simulink model "quad_control_elev8_attit_training"  (Simulink 8.7)
settings: Solver=FixedStepAuto  StartTime=0.0  StopTime=10  FixedStep=0.01  RelTol=1e-3
InitFcn:
  | % --- Inner loop gains --------
  | %Kp_pitch= 2.5; I_pitch =0.005; D_pitch = 0.5;
  | %Kp_roll = 2.5; I_roll =0.005; D_roll = 0.5;
  | %Kp_yaw = 10; I_yaw = 0.003; D_yaw = 2;
  | % --------------------------
  | 
  | % --- Outer loop gains --------
  | P_Z = 26.3889;
  | I_Z = 22.8237;
  | D_Z = 20.4994;
  | % --------------------------
  | 
  | % --- Saturation limits --------
  | mvel_upper_limit = 50;
  | mvel_lower_limit = 0;
  | % --------------------------
  | 
  | global clientID;
  | clientID=-1;
values from neighbouring files (symbols this model uses):
  D_pitch = 0.883609617998    [workspace_inner.mat]
  D_roll = 0.689579833659    [workspace_inner.mat]
  D_yaw = 2.7680176295    [workspace_inner.mat]
  I_pitch = 0.0103644908387    [workspace_inner.mat]
  I_roll = 0.00715888678063    [workspace_inner.mat]
  I_yaw = 0.00215447703315    [workspace_inner.mat]
  Kp_pitch = 3.99957984924    [workspace_inner.mat]
  Kp_roll = 4.19505963961    [workspace_inner.mat]
  Kp_yaw = 8.12783574482    [workspace_inner.mat]
undefined symbols (not defined in the file or in its folder): Angular, Linear
libraries: robotlib x7, simulink_extras x6, aerolibtransform2 x2
settings Model: Creator=kleber  LastModifiedBy=kleber
settings DebuggingCC: UnderspecifiedInitializationDetection=Simplified  MergeDetectMultiDrivingBlocksExec=error  SolverPrmCheckMsg=warning
settings ConfigComp: CovSFcnEnable=off

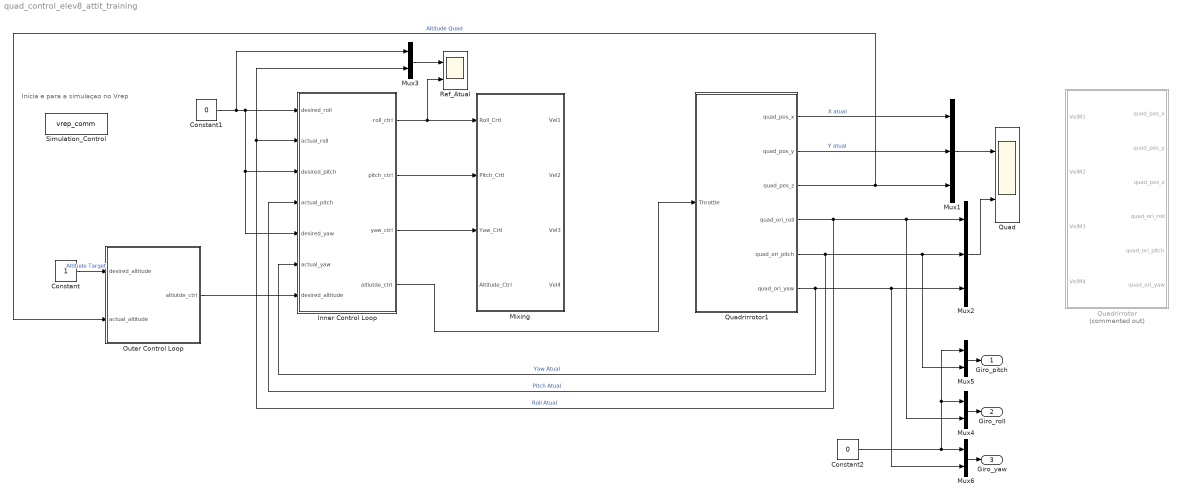
== system quad_control_elev8_attit_training ==
  note: Inicia e para a simulaçao no Vrep
  Constant : Constant
  Constant1 : Constant  Value=0
  Constant2 : Constant  Value=0
  Inner Control Loop : Subsystem
  Mixing : Subsystem
  Mux1 : Mux  Inputs=3
  Mux2 : Mux  Inputs=3
  Mux{3..6} (4 alike) : Mux  Inputs=2
  Outer Control Loop : Subsystem
  Quad : Scope  NumInputPorts=2
  Quadrirrotor : Subsystem  Commented=on
  Quadrirrotor1 : Subsystem
  Ref_Atual : Scope  NumInputPorts=2
  Simulation_Control : S-Function  FunctionName=vrep_comm  SFunctionDeploymentMode=off  EnableBusSupport=off
  Giro_pitch : Outport
  Giro_roll : Outport  Port=2
  Giro_yaw : Outport  Port=3
  wires:
  Mux1/1 -> Quad/1
  Mux2/1 -> Quad/2
  Quadrirrotor1/5(quad_ori_pitch) -> Mux2/2, Mux5/2, Inner Control Loop/4(actual_pitch)  "Pitch Atual"
  Quadrirrotor1/4(quad_ori_roll) -> Mux2/1, Mux4/2, Inner Control Loop/2(actual_roll), Mux3/2  "Roll Atual"
  Quadrirrotor1/1(quad_pos_x) -> Mux1/1  "X atual"
  Quadrirrotor1/3(quad_pos_z) -> Mux1/3, Outer Control Loop/2(actual_altitude)  "Altitude Quad"
  Quadrirrotor1/6(quad_ori_yaw) -> Mux6/2, Mux2/3, Inner Control Loop/6(actual_yaw)  "Yaw Atual"
  Inner Control Loop/4(altiutde_ctrl) -> Quadrirrotor1/1(Throttle)
  Constant1/1 -> Inner Control Loop/1(desired_roll), Inner Control Loop/5(desired_yaw), Inner Control Loop/3(desired_pitch), Mux3/1
  Outer Control Loop/1(altiutde_ctrl) -> Inner Control Loop/7(desired_altitude)
  Quadrirrotor1/2(quad_pos_y) -> Mux1/2  "Y atual"
  Constant/1 -> Outer Control Loop/1(desired_altitude)  "Altitude Target"
  Mux3/1 -> Ref_Atual/1
  Mux4/1 -> Giro_roll/1
  Mux5/1 -> Giro_pitch/1
  Mux6/1 -> Giro_yaw/1
  Constant2/1 -> Mux6/1, Mux4/1, Mux5/1
  Inner Control Loop/1(roll_ctrl) -> Ref_Atual/2, Mixing/1(Roll_Crtl)
  Inner Control Loop/2(pitch_ctrl) -> Mixing/2(Pitch_Crtl)
  Inner Control Loop/3(yaw_ctrl) -> Mixing/3(Yaw_Crtl)

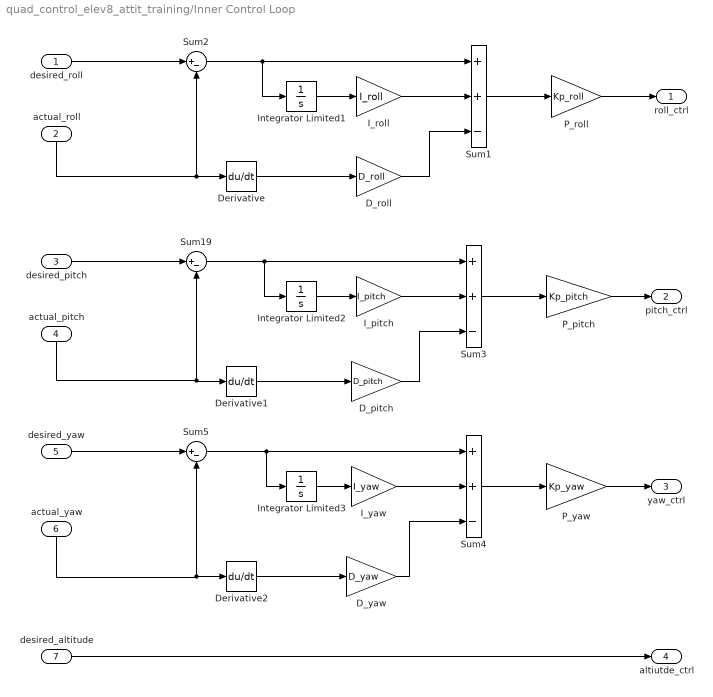
== system quad_control_elev8_attit_training/Inner Control Loop ==
  desired_roll : Inport
  actual_roll : Inport  Port=2
  desired_pitch : Inport  Port=3
  actual_pitch : Inport  Port=4
  desired_yaw : Inport  Port=5
  actual_yaw : Inport  Port=6
  desired_altitude : Inport  Port=7
  D_pitch : Gain  Gain=D_pitch
  D_roll : Gain  Gain=D_roll
  D_yaw : Gain  Gain=D_yaw
  Derivative : Derivative
  Derivative1 : Derivative
  Derivative2 : Derivative
  I_pitch : Gain  Gain=I_pitch
  I_roll : Gain  Gain=I_roll
  I_yaw : Gain  Gain=I_yaw
  Integrator Limited1 : Integrator  LimitOutput=on  UpperSaturationLimit=100  LowerSaturationLimit=-100
  Integrator Limited2 : Integrator  LimitOutput=on  UpperSaturationLimit=100  LowerSaturationLimit=-100
  Integrator Limited3 : Integrator  LimitOutput=on  UpperSaturationLimit=100  LowerSaturationLimit=-100
  P_pitch : Gain  Gain=Kp_pitch
  P_roll : Gain  Gain=Kp_roll
  P_yaw : Gain  Gain=Kp_yaw
  Sum1 : Sum  Inputs=++-
  Sum19 : Sum  Inputs=|+-
  Sum2 : Sum  Inputs=|+-
  Sum3 : Sum  Inputs=++-
  Sum4 : Sum  Inputs=++-
  Sum5 : Sum  Inputs=|+-
  roll_ctrl : Outport
  pitch_ctrl : Outport  Port=2
  yaw_ctrl : Outport  Port=3
  altiutde_ctrl : Outport  Port=4
  wires:
  desired_altitude/1 -> altiutde_ctrl/1
  Sum3/1 -> P_pitch/1
  P_pitch/1 -> pitch_ctrl/1
  D_pitch/1 -> Sum3/3
  Derivative1/1 -> D_pitch/1
  actual_pitch/1 -> Sum19/2, Derivative1/1
  Sum2/1 -> Integrator Limited1/1, Sum1/1
  Sum1/1 -> P_roll/1
  D_roll/1 -> Sum1/3
  Derivative/1 -> D_roll/1
  desired_pitch/1 -> Sum19/1
  actual_roll/1 -> Sum2/2, Derivative/1
  desired_roll/1 -> Sum2/1
  actual_yaw/1 -> Sum5/2, Derivative2/1
  Derivative2/1 -> D_yaw/1
  D_yaw/1 -> Sum4/3
  desired_yaw/1 -> Sum5/1
  P_roll/1 -> roll_ctrl/1
  P_yaw/1 -> yaw_ctrl/1
  I_roll/1 -> Sum1/2
  Sum19/1 -> Integrator Limited2/1, Sum3/1
  I_pitch/1 -> Sum3/2
  Sum4/1 -> P_yaw/1
  I_yaw/1 -> Sum4/2
  Integrator Limited2/1 -> I_pitch/1
  Integrator Limited1/1 -> I_roll/1
  Integrator Limited3/1 -> I_yaw/1
  Sum5/1 -> Integrator Limited3/1, Sum4/1

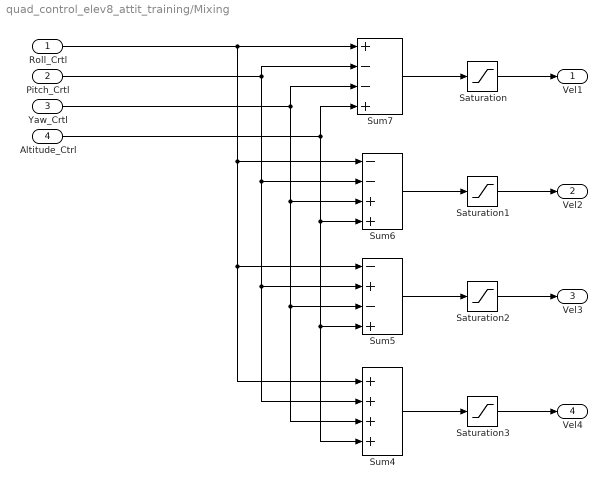
== system quad_control_elev8_attit_training/Mixing ==
  Roll_Crtl : Inport
  Pitch_Crtl : Inport  Port=2
  Yaw_Crtl : Inport  Port=3
  Altitude_Ctrl : Inport  Port=4
  Saturation{,1..3} (4 alike) : Saturate  UpperLimit=mvel_upper_limit  LowerLimit=mvel_lower_limit
  Sum4 : Sum  Inputs=++++
  Sum5 : Sum  Inputs=-+-+
  Sum6 : Sum  Inputs=--++
  Sum7 : Sum  Inputs=+--+
  Vel1 : Outport
  Vel2 : Outport  Port=2
  Vel3 : Outport  Port=3
  Vel4 : Outport  Port=4
  wires:
  Yaw_Crtl/1 -> Sum4/3, Sum5/3, Sum6/3, Sum7/3
  Roll_Crtl/1 -> Sum4/1, Sum5/1, Sum6/1, Sum7/1
  Pitch_Crtl/1 -> Sum4/2, Sum5/2, Sum6/2, Sum7/2
  Altitude_Ctrl/1 -> Sum4/4, Sum5/4, Sum6/4, Sum7/4
  Sum7/1 -> Saturation/1
  Saturation/1 -> Vel1/1
  Sum6/1 -> Saturation1/1
  Saturation1/1 -> Vel2/1
  Sum5/1 -> Saturation2/1
  Saturation2/1 -> Vel3/1
  Sum4/1 -> Saturation3/1
  Saturation3/1 -> Vel4/1

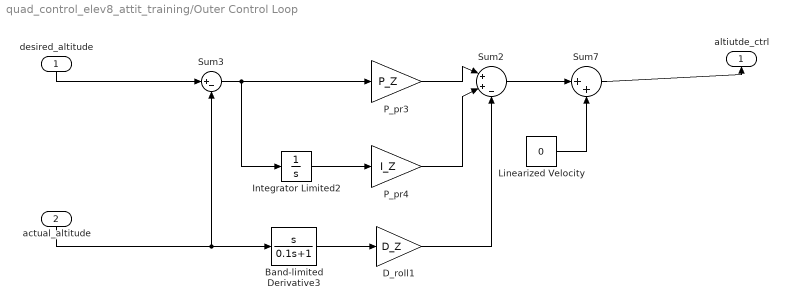
== system quad_control_elev8_attit_training/Outer Control Loop ==
  desired_altitude : Inport
  actual_altitude : Inport  Port=2
  Band-limited Derivative3 : TransferFcn  Numerator=[1 0]  Denominator=[0.1 1]
  D_roll1 : Gain  Gain=D_Z
  Integrator Limited2 : Integrator  LimitOutput=on  UpperSaturationLimit=5  LowerSaturationLimit=0
  Linearized Velocity : Constant  Value=0
  P_pr3 : Gain  Gain=P_Z
  P_pr4 : Gain  Gain=I_Z
  Sum2 : Sum  Inputs=|++-
  Sum3 : Sum  Inputs=|+-
  Sum7 : Sum  Inputs=|++
  altiutde_ctrl : Outport
  wires:
  Sum3/1 -> Integrator Limited2/1, P_pr3/1
  Integrator Limited2/1 -> P_pr4/1
  P_pr3/1 -> Sum2/1
  P_pr4/1 -> Sum2/2
  D_roll1/1 -> Sum2/3
  actual_altitude/1 -> Sum3/2, Band-limited Derivative3/1
  Band-limited Derivative3/1 -> D_roll1/1
  Sum2/1 -> Sum7/1
  Linearized Velocity/1 -> Sum7/2
  desired_altitude/1 -> Sum3/1
  Sum7/1 -> altiutde_ctrl/1

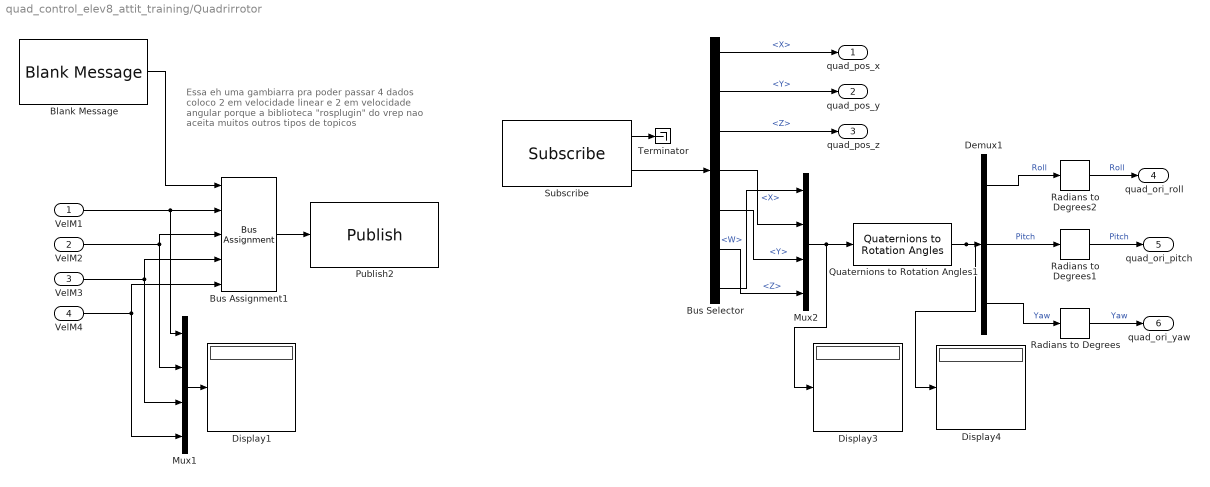
== system quad_control_elev8_attit_training/Quadrirrotor ==
  note: Essa eh uma gambiarra pra poder passar 4 dados coloco 2 em velocidade linear e 2 em velocidade angular porque a biblioteca "rosplugin" do vrep nao aceita muitos outros tipos de topicos
  VelM1 : Inport
  VelM2 : Inport  Port=2
  VelM3 : Inport  Port=3
  VelM4 : Inport  Port=4
  Blank Message : robotlib/Blank Message  SourceLibraryInfo=This block requires Robotics System Toolbox  messageType=geometry_msgs/Twist  SampleTime=inf
  Bus Assignment1 : BusAssignment  DialogController=Simulink.DDGSource_BusAssignment  AssignedSignals=Linear.X,Linear.Y,Angular.X,Angular.Y
  Bus Selector : BusSelector  OutputSignals=Pose.Position.X,Pose.Position.Y,Pose.Position.Z,Pose.Orientation.X,Pose.Orientation.Y,Pose.Orientation.Z,Pose.Orientation.W
  Demux1 : Demux  Outputs=3
  Display1 : Display
  Display3 : Display
  Display4 : Display
  Mux1 : Mux
  Mux2 : Mux
  Publish2 : robotlib/Publish  SourceLibraryInfo=This block requires Robotics System Toolbox  topicSource=Select from ROS network  topic=/motor_velocities  messageType=geometry_msgs/Twist  messageQueueLength=105
  Quaternions to Rotation Angles1 : aerolibtransform2/Quaternions to Rotation Angles  rotationOrder=XYZ
  Radians to Degrees : simulink_extras/Transformations/Radians to Degrees
  Radians to Degrees1 : simulink_extras/Transformations/Radians to Degrees
  Radians to Degrees2 : simulink_extras/Transformations/Radians to Degrees
  Subscribe : robotlib/Subscribe  SourceLibraryInfo=This block requires Robotics System Toolbox  topicSource=Select from ROS network  topic=/quad_pos_ang  messageType=geometry_msgs/PoseStamped  sampleTime=-1  messageQueueLength=51
  Terminator : Terminator
  quad_pos_x : Outport
  quad_pos_y : Outport  Port=2
  quad_pos_z : Outport  Port=3
  quad_ori_roll : Outport  Port=4
  quad_ori_pitch : Outport  Port=5
  quad_ori_yaw : Outport  Port=6
  wires:
  VelM1/1 -> Mux1/1, Bus Assignment1/2
  Bus Selector/1 -> quad_pos_x/1  "<X>"
  Bus Selector/2 -> quad_pos_y/1  "<Y>"
  Bus Selector/3 -> quad_pos_z/1  "<Z>"
  Radians to Degrees2/1 -> quad_ori_roll/1  "Roll"
  Radians to Degrees1/1 -> quad_ori_pitch/1  "Pitch"
  Radians to Degrees/1 -> quad_ori_yaw/1  "Yaw"
  Demux1/3 -> Radians to Degrees/1  "Yaw"
  Demux1/2 -> Radians to Degrees1/1  "Pitch"
  Demux1/1 -> Radians to Degrees2/1  "Roll"
  Bus Assignment1/1 -> Publish2/1
  Blank Message/1 -> Bus Assignment1/1
  Subscribe/2 -> Bus Selector/1
  Subscribe/1 -> Terminator/1
  Mux2/1 -> Quaternions to Rotation Angles1/1, Display3/1
  Bus Selector/5 -> Mux2/3  "<Y>"
  Bus Selector/6 -> Mux2/4  "<Z>"
  Bus Selector/7 -> Mux2/1  "<W>"
  Quaternions to Rotation Angles1/1 -> Demux1/1, Display4/1
  Bus Selector/4 -> Mux2/2  "<X>"
  VelM2/1 -> Bus Assignment1/3, Mux1/2
  VelM3/1 -> Bus Assignment1/4, Mux1/3
  VelM4/1 -> Bus Assignment1/5, Mux1/4
  Mux1/1 -> Display1/1

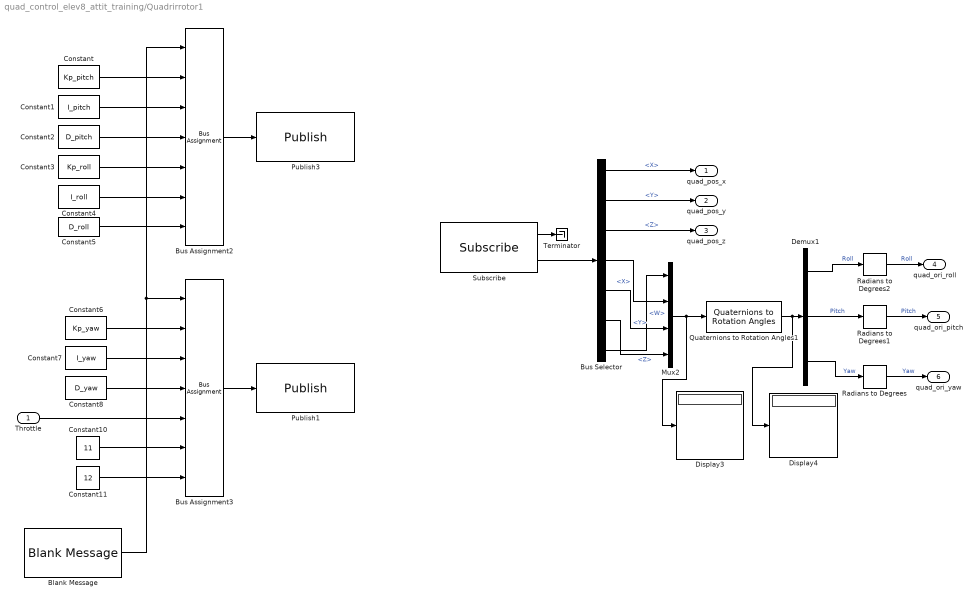
== system quad_control_elev8_attit_training/Quadrirrotor1 ==
  Throttle : Inport
  Blank Message : robotlib/Blank Message  SourceLibraryInfo=This block requires Robotics System Toolbox  messageType=geometry_msgs/Twist  SampleTime=inf
  Bus Assignment2 : BusAssignment  DialogController=Simulink.DDGSource_BusAssignment  AssignedSignals=Linear.X,Linear.Y,Linear.Z,Angular.X,Angular.Y,Angular.Z
  Bus Assignment3 : BusAssignment  DialogController=Simulink.DDGSource_BusAssignment  AssignedSignals=Linear.X,Linear.Y,Linear.Z,Angular.X,Angular.Y,Angular.Z
  Bus Selector : BusSelector  OutputSignals=Pose.Position.X,Pose.Position.Y,Pose.Position.Z,Pose.Orientation.X,Pose.Orientation.Y,Pose.Orientation.Z,Pose.Orientation.W
  Constant : Constant  Value=Kp_pitch
  Constant1 : Constant  Value=I_pitch
  Constant10 : Constant  Value=11
  Constant11 : Constant  Value=12
  Constant2 : Constant  Value=D_pitch
  Constant3 : Constant  Value=Kp_roll
  Constant4 : Constant  Value=I_roll
  Constant5 : Constant  Value=D_roll
  Constant6 : Constant  Value=Kp_yaw
  Constant7 : Constant  Value=I_yaw
  Constant8 : Constant  Value=D_yaw
  Demux1 : Demux  Outputs=3
  Display3 : Display
  Display4 : Display
  Mux2 : Mux
  Publish1 : robotlib/Publish  SourceLibraryInfo=This block requires Robotics System Toolbox  topicSource=Select from ROS network  topic=/gains2  messageType=geometry_msgs/Twist  messageQueueLength=105
  Publish3 : robotlib/Publish  SourceLibraryInfo=This block requires Robotics System Toolbox  topicSource=Select from ROS network  topic=/gains1  messageType=geometry_msgs/Twist  messageQueueLength=105
  Quaternions to Rotation Angles1 : aerolibtransform2/Quaternions to Rotation Angles  rotationOrder=XYZ
  Radians to Degrees : simulink_extras/Transformations/Radians to Degrees
  Radians to Degrees1 : simulink_extras/Transformations/Radians to Degrees
  Radians to Degrees2 : simulink_extras/Transformations/Radians to Degrees
  Subscribe : robotlib/Subscribe  SourceLibraryInfo=This block requires Robotics System Toolbox  topicSource=Select from ROS network  topic=/quad_pos_ang  messageType=geometry_msgs/PoseStamped  sampleTime=-1  messageQueueLength=51
  Terminator : Terminator
  quad_pos_x : Outport
  quad_pos_y : Outport  Port=2
  quad_pos_z : Outport  Port=3
  quad_ori_roll : Outport  Port=4
  quad_ori_pitch : Outport  Port=5
  quad_ori_yaw : Outport  Port=6
  wires:
  Bus Selector/1 -> quad_pos_x/1  "<X>"
  Bus Selector/2 -> quad_pos_y/1  "<Y>"
  Bus Selector/3 -> quad_pos_z/1  "<Z>"
  Radians to Degrees2/1 -> quad_ori_roll/1  "Roll"
  Radians to Degrees1/1 -> quad_ori_pitch/1  "Pitch"
  Radians to Degrees/1 -> quad_ori_yaw/1  "Yaw"
  Demux1/3 -> Radians to Degrees/1  "Yaw"
  Demux1/2 -> Radians to Degrees1/1  "Pitch"
  Demux1/1 -> Radians to Degrees2/1  "Roll"
  Blank Message/1 -> Bus Assignment3/1, Bus Assignment2/1
  Subscribe/2 -> Bus Selector/1
  Subscribe/1 -> Terminator/1
  Bus Selector/5 -> Mux2/3  "<Y>"
  Bus Selector/6 -> Mux2/4  "<Z>"
  Bus Selector/7 -> Mux2/1  "<W>"
  Mux2/1 -> Quaternions to Rotation Angles1/1, Display3/1
  Bus Selector/4 -> Mux2/2  "<X>"
  Quaternions to Rotation Angles1/1 -> Display4/1, Demux1/1
  Bus Assignment2/1 -> Publish3/1
  Constant/1 -> Bus Assignment2/2
  Constant1/1 -> Bus Assignment2/3
  Constant2/1 -> Bus Assignment2/4
  Constant3/1 -> Bus Assignment2/5
  Constant4/1 -> Bus Assignment2/6
  Bus Assignment3/1 -> Publish1/1
  Constant5/1 -> Bus Assignment2/7
  Constant6/1 -> Bus Assignment3/2
  Constant7/1 -> Bus Assignment3/3
  Constant8/1 -> Bus Assignment3/4
  Throttle/1 -> Bus Assignment3/5
  Constant10/1 -> Bus Assignment3/6
  Constant11/1 -> Bus Assignment3/7
